simulink model "list2_question3_simulink"  (R2014a)
settings: Solver=ode45  StartTime=0.0  StopTime=10.0  RelTol=1e-3
values from neighbouring files (symbols this model uses):
  alpha = 2    [list2_question3.m]
settings Model: Creator=Andre  LastModifiedBy=Andre
settings DataIOCC: SignalLoggingSaveFormat=ModelDataLogs
settings OptimizationCC: ExpressionDepthLimit=2147483647
settings DebuggingCC: UnderspecifiedInitializationDetection=Classic  FcnCallInpInsideContextMsg=UseLocalSettings  StateNameClashWarn=warning
settings GRTTargetCC: CombineOutputUpdateFcns=off  GRTInterface=on

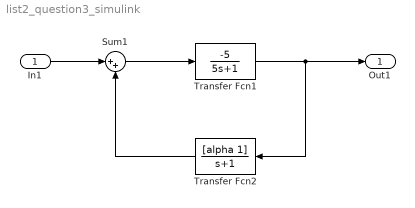
== system list2_question3_simulink ==
  In1 : Inport
  Sum1 : Sum  Inputs=|++
  Transfer Fcn1 : TransferFcn  Numerator=[-5]  Denominator=[5 1]
  Transfer Fcn2 : TransferFcn  Numerator=[alpha 1]  Denominator=[1 1]
  Out1 : Outport
  wires:
  Sum1/1 -> Transfer Fcn1/1
  Transfer Fcn1/1 -> Out1/1, Transfer Fcn2/1
  In1/1 -> Sum1/1
  Transfer Fcn2/1 -> Sum1/2
